simulink model "goodwin"  (R2024b)
settings: Solver=VariableStepAuto  StartTime=0.0  StopTime=tmax  MaxStep=1e-3
undefined symbols (not defined in the file): alpha, beta, delta, nu, phi0, phi1, x10, x20, y0
settings DataIOCC: ReturnWorkspaceOutputs=off

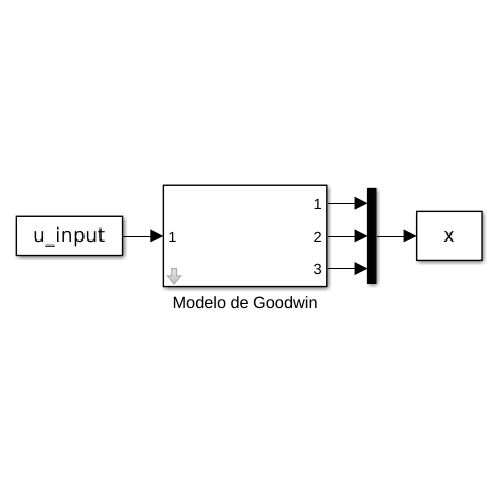
[thumbnail: Simulink's stored preview of the top-level diagram]
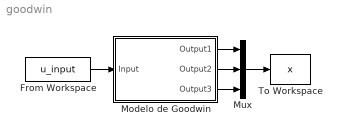
== system goodwin ==
  From Workspace : FromWorkspace  VariableName=u_input
  Modelo de Goodwin : Subsystem  mask(Modelo Goodwin){nu=nu, alpha=alpha, beta=beta, phi0=phi0, phi1=phi1, x0=[x10 x20]}
      mask prompts: x0 "c.i"
      mask help:
      | nu (ν): Tasa de capital a salida.
      | alpha (α): Tasa de crecimiento de la productividad.
      | beta (β): Tasa de crecimiento de la población.
      | delta (δ): Tasa de depreciación del capital.
      | phi1 (φ1) y phi0 (φ0): Parámetros de la curva de Phillips.
      mask Help:
      | Ecuaciones del modelo:
      | 
      | La tasa de cambio de x1 (proporción salarial) está dada por:
      | 
      | dx1/dt = x1 * [(phi1 / (1 - x2)^2) - phi0 - alpha]
      | Esto significa que la proporción salarial cambia en función del valor actual de la proporción salarial, el parámetro phi1, la tasa de empleo x2, el parámetro base phi0, y la tasa de crecimiento de la productividad alpha.
      | 
      | La tasa de cambio de x2 (tasa de empleo) está dada por:
      | 
      | dx2/dt = x2 * [(1 - x1) / nu - alpha - beta - delta] + u_input
      | Esto indica que la tasa de empleo cambia en función de su valor actual, la proporción salarial x1, el parámetro nu, la tasa de crecimiento de la productividad alpha, la tasa de crecimiento de la población beta, la tasa de depreciación del capital delta, y un factor externo representado por u_input.
      | 
      | La ecuación para la producción económica está dada por:
      | 
      | Y_output(t) = Y0 * (x2(t) / x2(0)) * exp((alpha + beta) * t)
      | Esto significa que la producción económica en el tiempo t depende del valor inicial de la producción Y0, la tasa de empleo en el tiempo t, la tasa de empleo inicial x2(0), y la combinación de las tasas de crecimiento de la productividad alpha y de la población beta.
  Mux : Mux  Inputs=3
  To Workspace : ToWorkspace  VariableName=x  SaveFormat=Structure With Time  SampleTime=-1
  wires:
  Mux/1 -> To Workspace/1
  From Workspace/1 -> Modelo de Goodwin/1(Input)
  Modelo de Goodwin/1(Output1) -> Mux/1
  Modelo de Goodwin/2(Output2) -> Mux/2
  Modelo de Goodwin/3(Output3) -> Mux/3

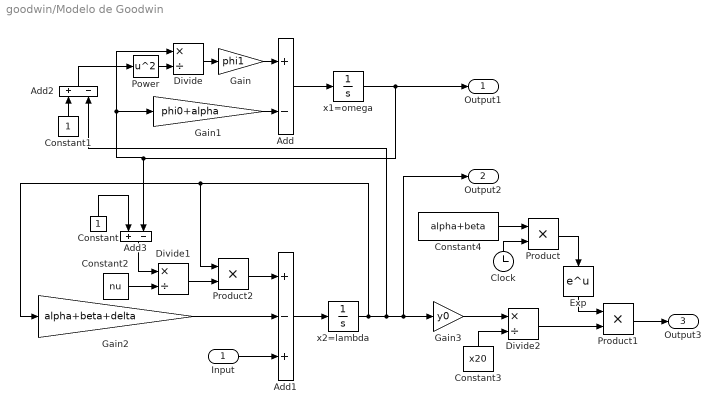
== system goodwin/Modelo de Goodwin ==
  Input : Inport
  Add : Sum  Inputs=+-
  Add1 : Sum  Inputs=+-+
  Add2 : Sum  Inputs=+-
  Add3 : Sum  Inputs=+-
  Clock : Clock
  Constant : Constant
  Constant1 : Constant
  Constant2 : Constant  Value=nu
  Constant3 : Constant  Value=x20
  Constant4 : Constant  Value=alpha+beta
  Divide : Product  Inputs=*/
  Divide1 : Product  Inputs=*/
  Divide2 : Product  Inputs=*/
  Exp : Math
  Gain : Gain  Gain=phi1
  Gain1 : Gain  Gain=phi0+alpha
  Gain2 : Gain  Gain=alpha+beta+delta
  Gain3 : Gain  Gain=y0
  Power : Math  Operator=square
  Product : Product
  Product1 : Product
  Product2 : Product
  x1=omega : Integrator  InitialCondition=x10
  x2=lambda : Integrator  InitialCondition=x20
  Output1 : Outport
  Output2 : Outport  Port=2
  Output3 : Outport  Port=3
  wires:
  Gain2/1 -> Add1/2
  Constant1/1 -> Add2/1
  Add/1 -> x1=omega/1
  x1=omega/1 -> Gain1/1, Divide/1, Add3/2, Output1/1
  Gain1/1 -> Add/2
  Add3/1 -> Divide1/1
  Add1/1 -> x2=lambda/1
  x2=lambda/1 -> Output2/1, Gain3/1, Add2/2, Gain2/1, Product2/1
  Constant/1 -> Add3/1
  Power/1 -> Divide/2
  Gain/1 -> Add/1
  Divide/1 -> Gain/1
  Constant2/1 -> Divide1/2
  Add2/1 -> Power/1
  Gain3/1 -> Divide2/1
  Constant3/1 -> Divide2/2
  Clock/1 -> Product/2
  Constant4/1 -> Product/1
  Product/1 -> Exp/1
  Exp/1 -> Product1/1
  Divide2/1 -> Product1/2
  Product1/1 -> Output3/1
  Input/1 -> Add1/3
  Divide1/1 -> Product2/2
  Product2/1 -> Add1/1
